simulink model "Husky_G2G"  (R2024b)
settings: Solver=VariableStepAuto  StartTime=0.0  StopTime=inf  RelTol=1e-3
settings Model: DataDictionary=DataDictionary.sldd  Creator=charber  LastModifiedBy=tsamak
settings ModelReferenceCC: ModelReferenceMinAlgLoopOccurrences=on

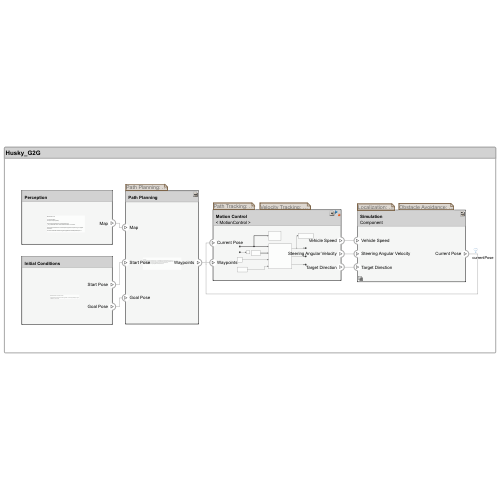
[thumbnail: Simulink's stored preview of the top-level diagram]
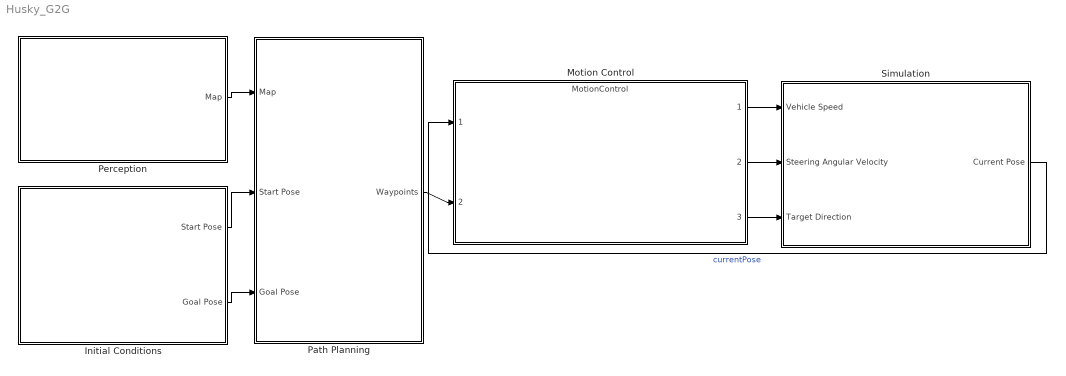
== system Husky_G2G ==
  Initial Conditions : Subsystem
      settings: PortSchema="{\"entries\":[{\"content\":{\"headerSize\":26,\"margin\":15,\"minimumSpacing\":25,\"sides\":[{\"content\":{},\"type\":\"ConnectorPlacement.EquallySpacedRectSide\",\"uuid\":\"8e0241d0-72c1-4096-95c2-f79012ec07cb\"},{\"content\":{\"connectorIds\":[\"Out1\",\"Out2\"],\"side\":\"RIGHT\"},\"type\":\"ConnectorPlacement.EquallySpacedRectSide\",\"uuid\":\"6de326a3-b92d-4bc0-b1e8-6032d07c2ebe\"},{\"content\":{\"side\":\"TOP\"},\"type\":\"ConnectorPlacement.EquallySpacedRectSide\",\"uuid\":\"3534b715-40a1-4058-baaf-53105771b364\"}]},\"type\":\"ConnectorPlacement.EquallySpacedConnector\",\"uuid\":\"09d1b855-ccea-4d7d-800b-1e4ad5961aa4\"}],\"packageUris\":[\"http://schema.mathworks.com/mf0/Connector/R2020b\"],\"version\":\"1.0\"}"
  Motion Control : ModelReference  ModelNameDialog=MotionControl  UsingDefaultArgumentValue=0,0  SimulationMode=Normal  ModelReferenceVersion=2.6
      settings: PortSchema="{\"entries\":[{\"content\":{\"headerSize\":38,\"margin\":15,\"minimumSpacing\":25,\"sides\":[{\"content\":{\"connectorIds\":[\"In1\",\"In2\"]},\"type\":\"ConnectorPlacement.EquallySpacedRectSide\",\"uuid\":\"c98b129e-902f-480e-b35c-0d51e818fc74\"},{\"content\":{\"connectorIds\":[\"Out1\",\"Out2\",\"Out3\"],\"side\":\"RIGHT\"},\"type\":\"ConnectorPlacement.EquallySpacedRectSide\",\"uuid\":\"6995c358-3616-4018-88cf-5d39b6da6a01\"},{\"content\":{\"side\":\"TOP\"},\"type\":\"ConnectorPlacement.EquallySpacedRectSide\",\"uuid\":\"9fd3bced-19a7-4eda-9800-31df169afecb\"}]},\"type\":\"ConnectorPlacement.EquallySpacedConnector\",\"uuid\":\"67565f83-f33b-4056-998b-9174ff38aca6\"}],\"packageUris\":[\"http://schema.mathworks.com/mf0/Connector/R2020b\"],\"version\":\"1.0\"}"
  Path Planning : Subsystem
      settings: PortSchema="{\"entries\":[{\"content\":{\"headerSize\":26,\"margin\":15,\"minimumSpacing\":25,\"sides\":[{\"content\":{\"connectorIds\":[\"In3\",\"In2\",\"In1\"]},\"type\":\"ConnectorPlacement.EquallySpacedRectSide\",\"uuid\":\"8e0241d0-72c1-4096-95c2-f79012ec07cb\"},{\"content\":{\"connectorIds\":[\"Out1\"],\"side\":\"RIGHT\"},\"type\":\"ConnectorPlacement.EquallySpacedRectSide\",\"uuid\":\"6de326a3-b92d-4bc0-b1e8-6032d07c2ebe\"},{\"content\":{\"side\":\"TOP\"},\"type\":\"ConnectorPlacement.EquallySpacedRectSide\",\"uuid\":\"3534b715-40a1-4058-baaf-53105771b364\"}]},\"type\":\"ConnectorPlacement.EquallySpacedConnector\",\"uuid\":\"09d1b855-ccea-4d7d-800b-1e4ad5961aa4\"}],\"packageUris\":[\"http://schema.mathworks.com/mf0/Connector/R2020b\"],\"version\":\"1.0\"}"
  Perception : Subsystem
      settings: PortSchema="{\"entries\":[{\"content\":{\"headerSize\":26,\"margin\":15,\"minimumSpacing\":25,\"sides\":[{\"content\":{},\"type\":\"ConnectorPlacement.EquallySpacedRectSide\",\"uuid\":\"8e0241d0-72c1-4096-95c2-f79012ec07cb\"},{\"content\":{\"connectorIds\":[\"Out1\"],\"side\":\"RIGHT\"},\"type\":\"ConnectorPlacement.EquallySpacedRectSide\",\"uuid\":\"6de326a3-b92d-4bc0-b1e8-6032d07c2ebe\"},{\"content\":{\"side\":\"TOP\"},\"type\":\"ConnectorPlacement.EquallySpacedRectSide\",\"uuid\":\"3534b715-40a1-4058-baaf-53105771b364\"}]},\"type\":\"ConnectorPlacement.EquallySpacedConnector\",\"uuid\":\"09d1b855-ccea-4d7d-800b-1e4ad5961aa4\"}],\"packageUris\":[\"http://schema.mathworks.com/mf0/Connector/R2020b\"],\"version\":\"1.0\"}"
  Simulation : Subsystem  Variant=on  VariantControlMode=label  LabelModeActiveChoice=Component
      settings: PortSchema="{\"entries\":[{\"content\":{\"headerSize\":38,\"margin\":15,\"minimumSpacing\":25,\"sides\":[{\"content\":{\"connectorIds\":[\"In2\",\"In3\",\"In1\"]},\"type\":\"ConnectorPlacement.EquallySpacedRectSide\",\"uuid\":\"928e42ed-4929-44d9-97ae-60c1add01b45\"},{\"content\":{\"connectorIds\":[\"Out1\"],\"side\":\"RIGHT\"},\"type\":\"ConnectorPlacement.EquallySpacedRectSide\",\"uuid\":\"265edb96-fe63-44e6-ab1f-9b35c7a83ccb\"},{\"content\":{\"side\":\"TOP\"},\"type\":\"ConnectorPlacement.EquallySpacedRectSide\",\"uuid\":\"c0006a31-ac86-4900-ae15-35bc44301cb7\"},{\"content\":{\"side\":\"BOTTOM\"},\"type\":\"ConnectorPlacement.EquallySpacedRectSide\",\"uuid\":\"3ee4aa34-6775-40d9-ae3d-040d6c8ae2c4\"}]},\"type\":\"ConnectorPlacement.EquallySpacedConnector\",\"uuid\":\"c5754a81-9857-403b-bbb7-4e4b912d146f\"}],\"packageUris\":[\"http://schema.mathworks.com/mf0/Connector/R2020b\"],\"version\":\"1.0\"}"
  wires:
  Initial Conditions/2(Goal Pose) -> Path Planning/1(Goal Pose)
  Initial Conditions/1(Start Pose) -> Path Planning/2(Start Pose)
  Perception/1(Map) -> Path Planning/3(Map)
  Simulation/1(Current Pose) -> Motion Control/1  "currentPose"
  Path Planning/1(Waypoints) -> Motion Control/2
  Motion Control/2 -> Simulation/3(Steering Angular Velocity)
  Motion Control/3 -> Simulation/1(Target Direction)
  Motion Control/1 -> Simulation/2(Vehicle Speed)

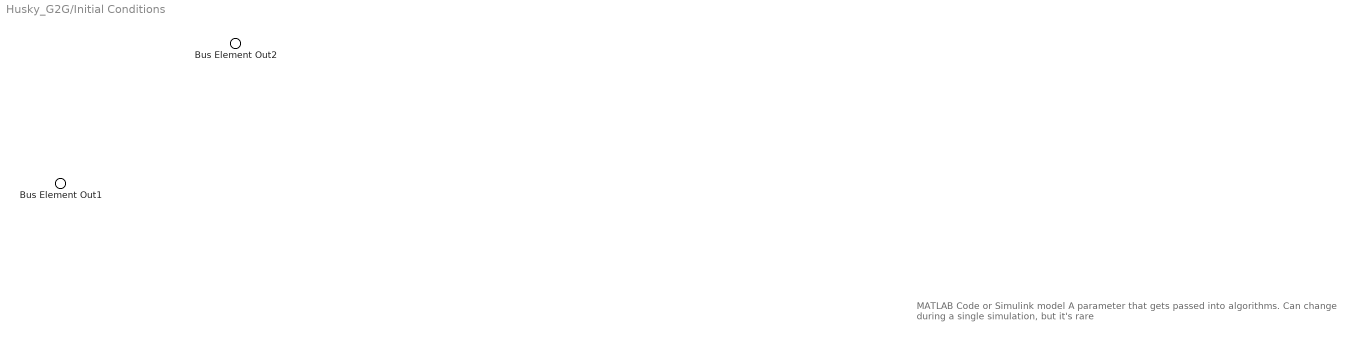
== system Husky_G2G/Initial Conditions ==
  note: MATLAB Code or Simulink model
      |
      | A parameter that gets passed into algorithms. Can change during a single simulation, but it's rare
  Bus Element Out2 : Outport  PortName=Start Pose
  Bus Element Out1 : Outport  Port=2  PortName=Goal Pose

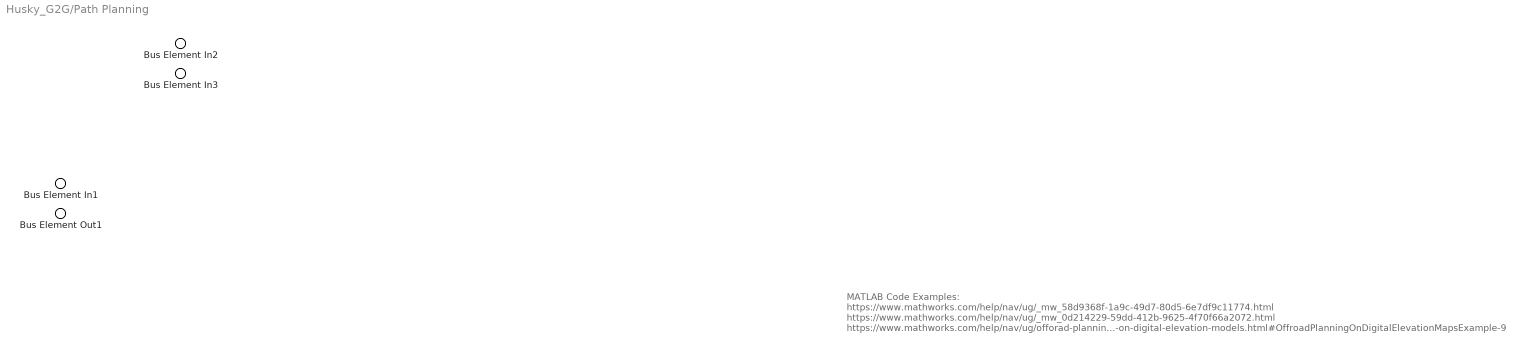
== system Husky_G2G/Path Planning ==
  note: MATLAB Code
      |
      | Examples:
      | https://www.mathworks.com/help/nav/ug/_mw_58d9368f-1a9c-49d7-80d5-6e7df9c11774.html
      | https://www.mathworks.com/help/nav/ug/_mw_0d214229-59dd-412b-9625-4f70f66a2072.html
      | https://www.mathworks.com/help/nav/ug/offorad-planning-on-digital-elevation-models.html#OffroadPlanningOnDigitalElevationMapsExample-9
  Bus Element In2 : Inport  PortName=Goal Pose
  Bus Element In3 : Inport  Port=2  PortName=Start Pose
  Bus Element In1 : Inport  Port=3  PortName=Map
  Bus Element Out1 : Outport  PortName=Waypoints

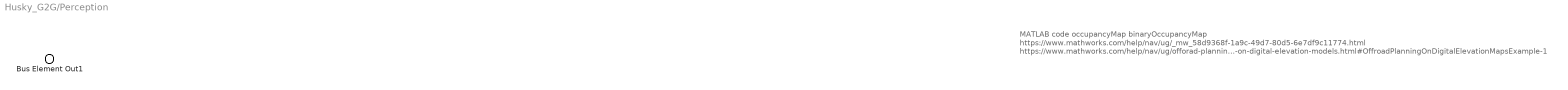
== system Husky_G2G/Perception ==
  note: MATLAB code
      |
      | occupancyMap
      | binaryOccupancyMap
      |
      | https://www.mathworks.com/help/nav/ug/_mw_58d9368f-1a9c-49d7-80d5-6e7df9c11774.html
      |
      | https://www.mathworks.com/help/nav/ug/offorad-planning-on-digital-elevation-models.html#OffroadPlanningOnDigitalElevationMapsExample-1
  Bus Element Out1 : Outport  PortName=Map

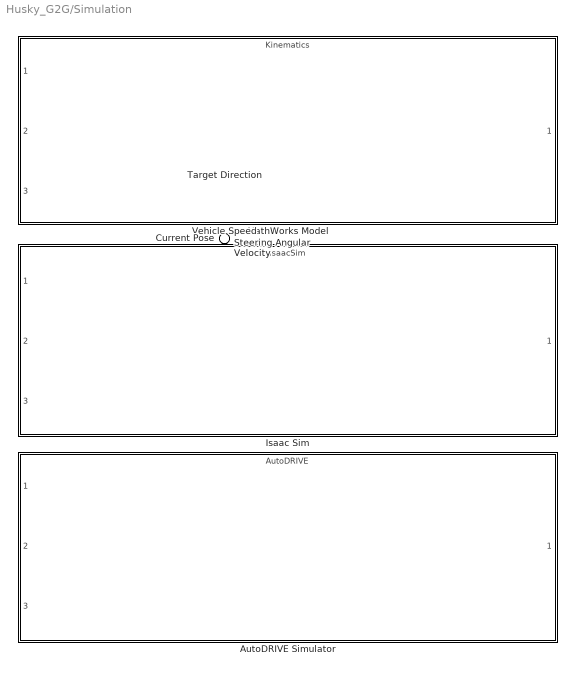
== system Husky_G2G/Simulation ==
  Target Direction : Inport
  Vehicle Speed : Inport  Port=2  OutDataTypeStr=double
  Steering Angular Velocity : Inport  Port=3  OutDataTypeStr=double
  AutoDRIVE Simulator : ModelReference  ModelNameDialog=AutoDRIVE  SimulationMode=Normal  VariantControl=Component  ModelReferenceVersion=1.21
      settings: PortSchema="{\"entries\":[{\"content\":{\"headerSize\":38,\"margin\":15,\"minimumSpacing\":25,\"sides\":[{\"content\":{\"connectorIds\":[\"In1\",\"In2\",\"In3\"]},\"type\":\"ConnectorPlacement.EquallySpacedRectSide\",\"uuid\":\"fff1038f-badb-4c3d-a9b4-39a003bde29c\"},{\"content\":{\"connectorIds\":[\"Out1\"],\"side\":\"RIGHT\"},\"type\":\"ConnectorPlacement.EquallySpacedRectSide\",\"uuid\":\"acfb8ae9-60f1-493f-9871-3959ae422a33\"},{\"content\":{\"side\":\"TOP\"},\"type\":\"ConnectorPlacement.EquallySpacedRectSide\",\"uuid\":\"e34f200b-c261-4832-b8dd-0cbae5258d3b\"}]},\"type\":\"ConnectorPlacement.EquallySpacedConnector\",\"uuid\":\"d4137258-0861-4dce-ac93-2c30ef95f038\"}],\"packageUris\":[\"http://schema.mathworks.com/mf0/Connector/R2020b\"],\"version\":\"1.0\"}"
  Isaac Sim : ModelReference  ModelNameDialog=IsaacSim  SimulationMode=Normal  VariantControl=IsaacSim  ModelReferenceVersion=2.1
      settings: PortSchema="{\"entries\":[{\"content\":{\"headerSize\":38,\"margin\":15,\"minimumSpacing\":25,\"sides\":[{\"content\":{\"connectorIds\":[\"In1\",\"In2\",\"In3\"]},\"type\":\"ConnectorPlacement.EquallySpacedRectSide\",\"uuid\":\"c98b129e-902f-480e-b35c-0d51e818fc74\"},{\"content\":{\"connectorIds\":[\"Out1\"],\"side\":\"RIGHT\"},\"type\":\"ConnectorPlacement.EquallySpacedRectSide\",\"uuid\":\"6995c358-3616-4018-88cf-5d39b6da6a01\"},{\"content\":{\"side\":\"TOP\"},\"type\":\"ConnectorPlacement.EquallySpacedRectSide\",\"uuid\":\"9fd3bced-19a7-4eda-9800-31df169afecb\"}]},\"type\":\"ConnectorPlacement.EquallySpacedConnector\",\"uuid\":\"67565f83-f33b-4056-998b-9174ff38aca6\"}],\"packageUris\":[\"http://schema.mathworks.com/mf0/Connector/R2020b\"],\"version\":\"1.0\"}"
  MathWorks Model : ModelReference  ModelNameDialog=Kinematics.slx  SimulationMode=Normal  VariantControl=MathWorksModel  ModelReferenceVersion=1.19
      settings: PortSchema="{\"entries\":[{\"content\":{\"headerSize\":38,\"margin\":15,\"minimumSpacing\":25,\"sides\":[{\"content\":{\"connectorIds\":[\"In1\",\"In2\",\"In3\"]},\"type\":\"ConnectorPlacement.EquallySpacedRectSide\",\"uuid\":\"c98b129e-902f-480e-b35c-0d51e818fc74\"},{\"content\":{\"connectorIds\":[\"Out1\"],\"side\":\"RIGHT\"},\"type\":\"ConnectorPlacement.EquallySpacedRectSide\",\"uuid\":\"6995c358-3616-4018-88cf-5d39b6da6a01\"},{\"content\":{\"side\":\"TOP\"},\"type\":\"ConnectorPlacement.EquallySpacedRectSide\",\"uuid\":\"9fd3bced-19a7-4eda-9800-31df169afecb\"}]},\"type\":\"ConnectorPlacement.EquallySpacedConnector\",\"uuid\":\"67565f83-f33b-4056-998b-9174ff38aca6\"}],\"packageUris\":[\"http://schema.mathworks.com/mf0/Connector/R2020b\"],\"version\":\"1.0\"}"
  Current Pose : Outport
